simulink model "AsynCnt3"  (R2025b)
settings: Solver=VariableStepAuto  StartTime=0.0  StopTime=Inf  RelTol=1e-3
settings Model: Creator=Soochan Kim  LastModifiedBy=Soochan Kim

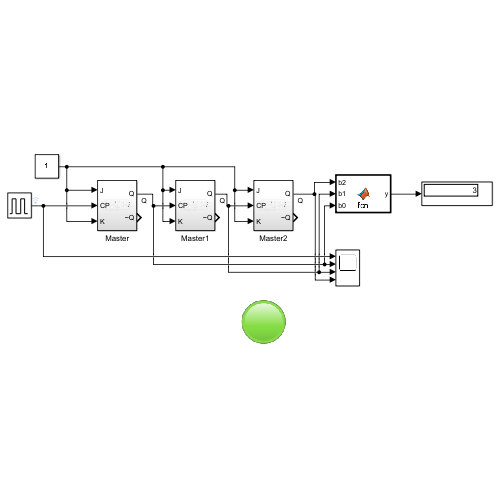
[thumbnail: Simulink's stored preview of the top-level diagram]
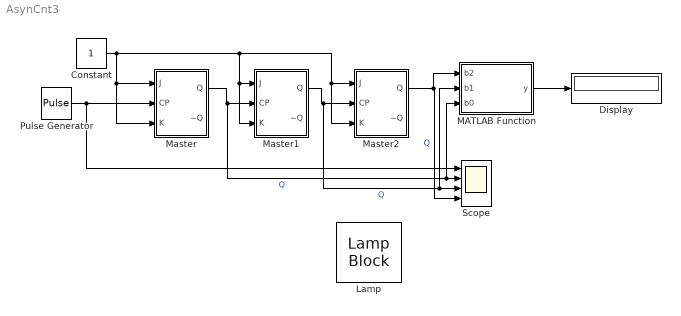
== system AsynCnt3 ==
  Constant : Constant
  Display : Display
  Lamp : LampBlock  LabelPosition=Hide  DefaultColor=[192.0, 192.0, 192.0]
  MATLAB Function : MATLAB Function  TreatAsAtomicUnit=on
  Master : Subsystem
  Master1 : Subsystem
  Master2 : Subsystem
  Pulse Generator : DiscretePulseGenerator  PulseType=Time based  Period=1  PulseWidth=50  PhaseDelay=0.5
  Scope : Scope  NumInputPorts=4
      settings: ActiveDisplayYMinimum=-0.12499999999999997  ActiveDisplayYMaximum=1.125
  wires:
  Constant/1 -> Master/3(K), Master/1(J), Master1/1(J), Master1/3(K), Master2/3(K), Master2/1(J)
  Pulse Generator/1 -> Scope/1, Master/2(CP)
  Master/1(Q) -> MATLAB Function/3(b0), Scope/2, Master1/2(CP)  "Q"
  Master1/1(Q) -> Master2/2(CP), MATLAB Function/2(b1), Scope/3  "Q"
  Master2/1(Q) -> MATLAB Function/1(b2), Scope/4  "Q"
  MATLAB Function/1(y) -> Display/1

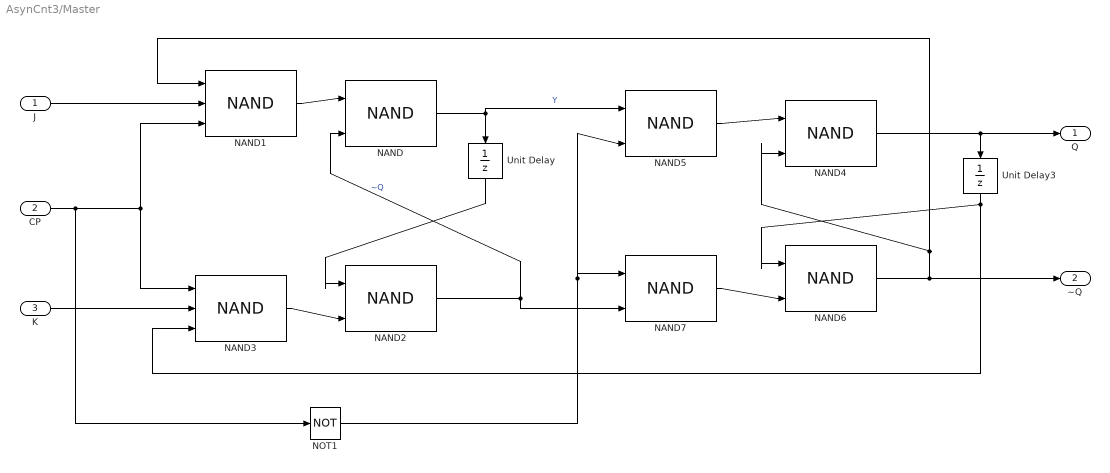
== system AsynCnt3/Master ==
  J : Inport
  CP : Inport  Port=2
  K : Inport  Port=3
  NAND{,2,4..7} (6 alike) : Logic  Operator=NAND  IconShape=distinctive  AllPortsSameDT=off  OutDataTypeStr=boolean
  NAND1 : Logic  Operator=NAND  Inputs=3  IconShape=distinctive  AllPortsSameDT=off  OutDataTypeStr=boolean
  NAND3 : Logic  Operator=NAND  Inputs=3  IconShape=distinctive  AllPortsSameDT=off  OutDataTypeStr=boolean
  NOT1 : Logic  Operator=NOT  IconShape=distinctive  AllPortsSameDT=off  OutDataTypeStr=boolean
  Unit Delay : UnitDelay  SampleTime=0.001  HasFrameUpgradeWarning=on
  Unit Delay3 : UnitDelay  SampleTime=-1  HasFrameUpgradeWarning=on
  Q : Outport
  ~Q : Outport  Port=2
  wires:
  NAND/1 -> Unit Delay/1, NAND5/1  "Y"
  NAND2/1 -> NAND/2, NAND7/2  "~Q"
  Unit Delay/1 -> NAND2/1
  K/1 -> NAND3/2
  NAND1/1 -> NAND/1
  NAND3/1 -> NAND2/2
  J/1 -> NAND1/2
  NAND6/1 -> ~Q/1, NAND1/1, NAND4/2
  Unit Delay3/1 -> NAND3/3, NAND6/1
  NAND5/1 -> NAND4/1
  NAND7/1 -> NAND6/2
  NAND4/1 -> Q/1, Unit Delay3/1
  CP/1 -> NAND3/1, NAND1/3, NOT1/1
  NOT1/1 -> NAND5/2, NAND7/1

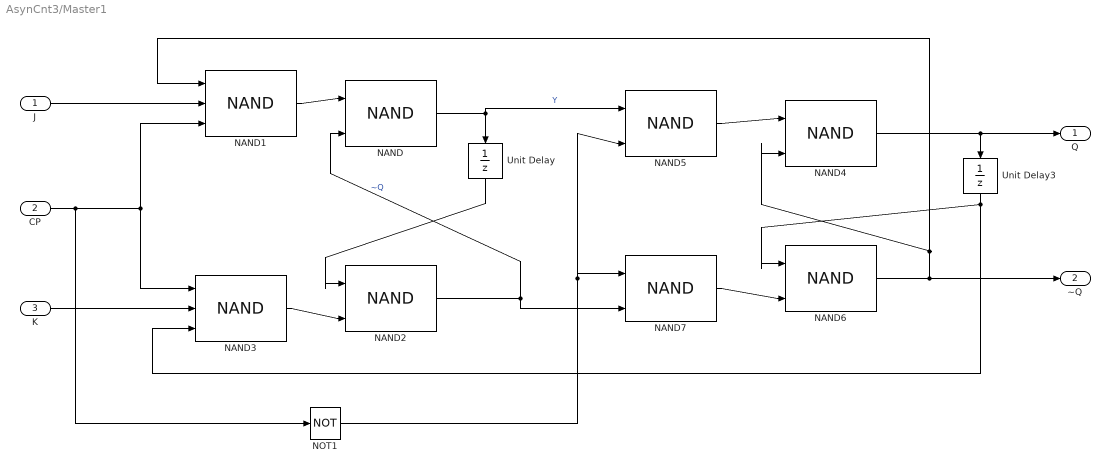
== system AsynCnt3/Master1 ==
  J : Inport
  CP : Inport  Port=2
  K : Inport  Port=3
  NAND{,2,4..7} (6 alike) : Logic  Operator=NAND  IconShape=distinctive  AllPortsSameDT=off  OutDataTypeStr=boolean
  NAND1 : Logic  Operator=NAND  Inputs=3  IconShape=distinctive  AllPortsSameDT=off  OutDataTypeStr=boolean
  NAND3 : Logic  Operator=NAND  Inputs=3  IconShape=distinctive  AllPortsSameDT=off  OutDataTypeStr=boolean
  NOT1 : Logic  Operator=NOT  IconShape=distinctive  AllPortsSameDT=off  OutDataTypeStr=boolean
  Unit Delay : UnitDelay  SampleTime=0.001  HasFrameUpgradeWarning=on
  Unit Delay3 : UnitDelay  SampleTime=-1  HasFrameUpgradeWarning=on
  Q : Outport
  ~Q : Outport  Port=2
  wires:
  NAND/1 -> Unit Delay/1, NAND5/1  "Y"
  NAND2/1 -> NAND/2, NAND7/2  "~Q"
  Unit Delay/1 -> NAND2/1
  K/1 -> NAND3/2
  NAND1/1 -> NAND/1
  NAND3/1 -> NAND2/2
  J/1 -> NAND1/2
  NAND6/1 -> ~Q/1, NAND1/1, NAND4/2
  Unit Delay3/1 -> NAND3/3, NAND6/1
  NAND5/1 -> NAND4/1
  NAND7/1 -> NAND6/2
  NAND4/1 -> Q/1, Unit Delay3/1
  CP/1 -> NAND3/1, NAND1/3, NOT1/1
  NOT1/1 -> NAND5/2, NAND7/1

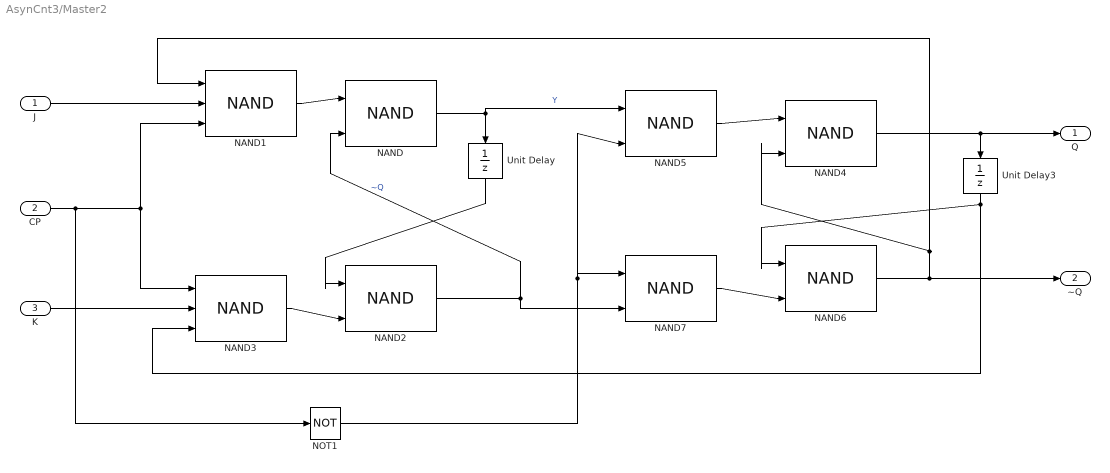
== system AsynCnt3/Master2 ==
  J : Inport
  CP : Inport  Port=2
  K : Inport  Port=3
  NAND{,2,4..7} (6 alike) : Logic  Operator=NAND  IconShape=distinctive  AllPortsSameDT=off  OutDataTypeStr=boolean
  NAND1 : Logic  Operator=NAND  Inputs=3  IconShape=distinctive  AllPortsSameDT=off  OutDataTypeStr=boolean
  NAND3 : Logic  Operator=NAND  Inputs=3  IconShape=distinctive  AllPortsSameDT=off  OutDataTypeStr=boolean
  NOT1 : Logic  Operator=NOT  IconShape=distinctive  AllPortsSameDT=off  OutDataTypeStr=boolean
  Unit Delay : UnitDelay  SampleTime=0.001  HasFrameUpgradeWarning=on
  Unit Delay3 : UnitDelay  SampleTime=-1  HasFrameUpgradeWarning=on
  Q : Outport
  ~Q : Outport  Port=2
  wires:
  NAND/1 -> Unit Delay/1, NAND5/1  "Y"
  NAND2/1 -> NAND/2, NAND7/2  "~Q"
  Unit Delay/1 -> NAND2/1
  K/1 -> NAND3/2
  NAND1/1 -> NAND/1
  NAND3/1 -> NAND2/2
  J/1 -> NAND1/2
  NAND6/1 -> ~Q/1, NAND1/1, NAND4/2
  Unit Delay3/1 -> NAND3/3, NAND6/1
  NAND5/1 -> NAND4/1
  NAND7/1 -> NAND6/2
  NAND4/1 -> Q/1, Unit Delay3/1
  CP/1 -> NAND3/1, NAND1/3, NOT1/1
  NOT1/1 -> NAND5/2, NAND7/1

== matlab function AsynCnt3/MATLAB Function ==
  data: b2 input; y output; b1 input; b0 input
function y = fcn(b2, b1, b0)

u= b2*4 + b1*2 + b0*1;

y = u;
end
